simulink model "trabalho3_controle_digital2023"  (R2023a)
settings: Solver=VariableStepAuto  StartTime=0.0  StopTime=20  RelTol=1e-6
settings Model: LastModifiedBy=DELL
settings RTWCC: GPUComputeCapability=5.0

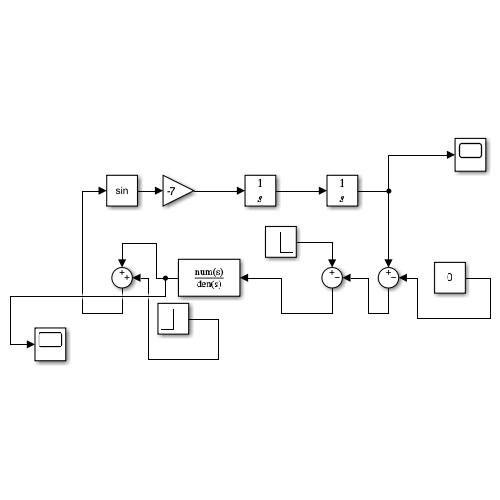
[thumbnail: Simulink's stored preview of the top-level diagram]
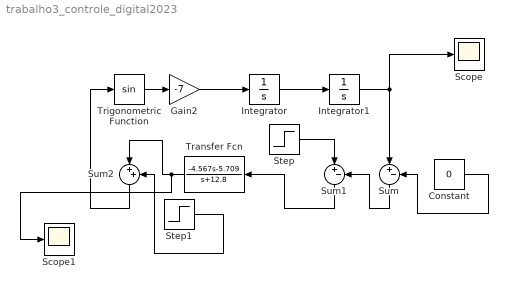
== system trabalho3_controle_digital2023 ==
  Constant : Constant  Value=0
  Gain2 : Gain  Gain=-7
  Integrator : Integrator
  Integrator1 : Integrator
  Scope : Scope
  Scope1 : Scope
  Step : Step  After=-0.5  SampleTime=0
  Step1 : Step  Time=5  After=0.05  SampleTime=0
  Sum : Sum  Inputs=|+-
  Sum1 : Sum  Inputs=|+-
  Sum2 : Sum  Inputs=|++
  Transfer Fcn : TransferFcn  Numerator=[-4.567 -5.709]  Denominator=[1 12.8]
  Trigonometric Function : Trigonometry
  wires:
  Integrator/1 -> Integrator1/1
  Trigonometric Function/1 -> Gain2/1
  Gain2/1 -> Integrator/1
  Integrator1/1 -> Scope/1, Sum/1
  Constant/1 -> Sum/2
  Sum/1 -> Sum1/2
  Step/1 -> Sum1/1
  Sum1/1 -> Transfer Fcn/1
  Transfer Fcn/1 -> Scope1/1, Sum2/1
  Sum2/1 -> Trigonometric Function/1
  Step1/1 -> Sum2/2
